simulink model "PMS_Motor_level2"  (Simulink 6.4)
settings: Solver=FixedStepDiscrete  StartTime=0.0  StopTime=0.3  RelTol=1e-3
values from neighbouring files (symbols this model uses):
  DC_voltage = 200    [PMS_Motor_data.m]
  model = 'AM_Sqrt'    [ChangeModel.m]    (also in SelectModel.m = 'MCov_AR')
  Ts = 5e-5    (= 5e-05)    [PMS_Motor_data.m]
libraries: powerlib x12, c28xdmclib x4, simulink x4, tiiqmathlib x3, c281xdspchiplib x2, c2000tgtpreflib x1, powerlib_extras x1
CloseFcn:
  | rtwprivate ssgencode ModelCloseRequest Simple_DC_Motor
settings Model: LastModifiedBy=greith  ProdHWDeviceType=TI C2000
settings DataIOCC: SaveOutput=off  SaveTime=off  SignalLoggingName=DataLog
settings OptimizationCC: OptimizeModelRefInitCode=on  LifeSpan=1
settings DebuggingCC: ReadBeforeWriteMsg=DisableAll  ParameterPrecisionLossMsg=none  StrictBusMsg=ErrorLevel1
settings HardwareCC: ProdBitPerChar=16  ProdBitPerInt=16  ProdIntDivRoundTo=Zero  ProdEndianess=LittleEndian  ProdWordSize=16  ProdHWDeviceType=TI C2000  TargetHWDeviceType=32-bit Generic
settings RTWCC: SystemTargetFile=ti_c2000_ert.tlc  GenCodeOnly=on  TemplateMakefile=ti_c2000_ert.tmf  Description=Embedded Target for TI C2000 DSP (ERT)  GenerateReport=on  ProcessScript=ti_c2000_ert_make_rtw_hook  IncludeHyperlinkInReport=on  LaunchReport=on
settings CodeAppCC: IgnoreCustomStorageClasses=off
settings STFCustomTargetCC: TargetFcnLib=ansi_tfl_tmw.mat  GenFloatMathFcnCalls=ANSI_C  ModelReferenceCompliant=off  CombineOutputUpdateFcns=on  IncludeERTFirstTime=on  ERTCustomFileBanners=on  SystemTargetFile=ti_c2000_ert.tlc
settings ERTTargetCC: TargetFcnLib=ansi_tfl_tmw.mat  GenFloatMathFcnCalls=ANSI_C  ModelReferenceCompliant=off  IncludeERTFirstTime=on  ERTFirstTimeCompliant=off  SupportContinuousTime=on  SupportNonInlinedSFcns=on  InlinedParameterPlacement=NonHierarchical  ERTCustomFileTemplate=example_file_process.tlc  InitialValueSource=Model

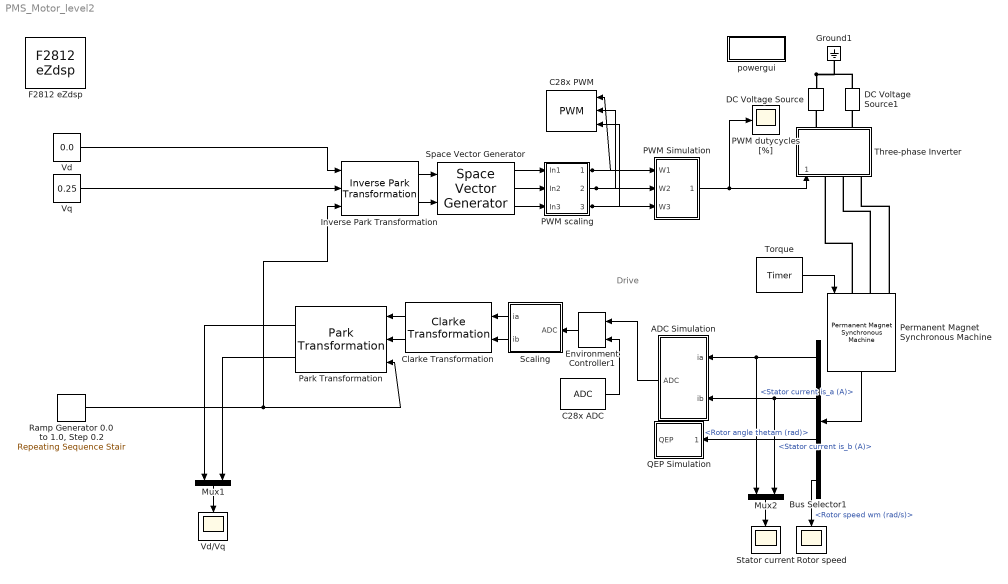
== system PMS_Motor_level2 ==
  note: Drive
  ADC Simulation : Subsystem  Orientation=left
  Bus Selector1 : BusSelector  Orientation=left  OutputSignals=Stator current is_a (A),Stator current is_b (A),Rotor angle thetam (rad),Rotor speed wm (rad/s)
  C28x ADC : c281xdspchiplib/ADC  useModule=A  useMode=Sequential  sourceSOC=Software  Ts=-1  dType=uint16  postInterrupt=off  numConversionsSingle=3  numConversionsDouble=1  conv0=ADCINB0  conv1=ADCINB1  conv2=ADCINB2  conv3=ADCINB3  conv4=ADCINA4  conv5=ADCINA5  conv6=ADCINB6  conv7=ADCINA7  conv8=ADCINB0  conv9=ADCINB1  conv10=ADCINB2  conv11=ADCINB3  conv12=ADCINB4  conv13=ADCINB5  conv14=ADCINB6  conv15=ADCINB7  convAB0=ADCINA0 and ADCINB0  convAB1=ADCINA1 and ADCINB1  convAB2=ADCINA5 and ADCINB5  convAB3=ADCINA1 and ADCINB1  convAB4=ADCINA1 and ADCINB1  convAB5=ADCINA1 and ADCINB1  convAB6=ADCINA1 and ADCINB1  convAB7=ADCINA1 and ADCINB1  convA0=ADCINA0  convA1=ADCINA1  convA2=ADCINA7  convA3=ADCINA3  convA4=ADCINA4  convA5=ADCINA5  convA6=ADCINA6  convA7=ADCINA7  convB0=ADCINB0  convB1=ADCINB1  convB2=ADCINB2  convB3=ADCINB3  convB4=ADCINB4  convB5=ADCINB5  convB6=ADCINB6  convB7=ADCINB7  c28xmultiPort=off
  C28x PWM : c281xdspchiplib/PWM  Orientation=left  useModule=A  timerSource=Specify via dialog  timerPeriod=(2^12)+1  waveformType=Symmetric  periodUnits=Clock cycles  unit1Status=on  unit1Source=Input port  unit1Value=4096  unit2Status=on  unit2Source=Input port  unit2Value=4096  unit3Status=on  unit3Source=Input port  unit3Value=4096  dutyCycleUnits=Clock cycles  logicSource=Specify via dialog  unit1_1Logic=Active high  unit1_2Logic=Active low  unit2_1Logic=Active high  unit2_2Logic=Active low  unit3_1Logic=Active high  unit3_2Logic=Active low  enableDeadband1=on  enableDeadband2=on  enableDeadband3=on  deadbandPrescaler=8  deadbandPeriodSource=Specify via dialog  deadbandPeriod=15  adcstartEvent=None
  Clarke Transformation : c28xdmclib/Clarke Transformation  Orientation=left
  DC Voltage Source : powerlib/Electrical Sources/DC Voltage Source  Orientation=down  SystemSampleTime=-1  Amplitude=DC_voltage  Measurements=None
  DC Voltage Source1 : powerlib/Electrical Sources/DC Voltage Source  Orientation=up  SystemSampleTime=-1  Amplitude=DC_voltage  Measurements=None
  Environment Controller1 : simulink/Signal Routing/Environment Controller  Orientation=left  SystemSampleTime=-1
  F2812 eZdsp : c2000tgtpreflib/F2812 eZdsp  Tag=C2000 TARGET PREFERENCES BLOCK  SystemSampleTime=-1
  Ground1 : powerlib/Elements/Ground  Orientation=up  PhysicalDomain=powersysdomain  SubClassName=unknown  LeftPortType=p1  RightPortType=p1  LConnTagsString=a
  Inverse Park Transformation : c28xdmclib/Inverse Park Transformation
  Mux1 : Mux  Orientation=down  Inputs=2
  Mux2 : Mux  Orientation=down  Inputs=2
  PWM Simulation : Subsystem
  PWM dutycycles [%] : Scope
      settings: TimeRange=1.8  YMin=0.35  YMax=0.625  SaveName=ScopeData4
  PWM scaling : Subsystem
  Park Transformation : c28xdmclib/Park Transformation  Orientation=left
  Permanent Magnet Synchronous Machine : powerlib/Machines/Permanent Magnet Synchronous Machine  Orientation=down  SystemSampleTime=-1  FluxDistribution=Sinusoidal  MechanicalLoad=Torque Tm  PresetModel=No  ShowDetailedParameters=on  Resistance=1.6  Inductance=8.5e-3  dqInductances=[0.006365 0.006365]  Flux=0.1852  Flat=120  Mechanical=[0.0001854 5.396e-005 1]
  QEP Simulation : Subsystem  Orientation=left
  "Ramp Generator 0.0 to 1.0, Step 0.2" : simulink/Sources/Repeating Sequence Stair  SystemSampleTime=-1  OutValues=[0.0:0.0005:1.0]  tsamp=0.00005  OutputDataTypeScalingMode=Specify via dialog  OutDataType=sfix(32)  ConRadixGroup=Use Specified Scaling  OutScaling=2^-17
  Rotor speed : Scope
      settings: Orientation=down  TimeRange=4.5  YMin=-150  YMax=1000
  Scaling : Subsystem  Orientation=left
  Space Vector Generator : c28xdmclib/Space Vector Generator
  Stator current : Scope
      settings: Orientation=down  TimeRange=0.5567010309278351  YMin=0  YMax=4000  SaveName=ScopeData6
  Three-phase Inverter : Subsystem  Orientation=up  AncestorBlock=AC2DriveInternalModels/Three-phase Inverter (average model)  mask(SPSdrives Converter){Device=IGBT / Diodes, SnubberResistance=500, SnubberCapacitance=1e-9, Ron=1e-3, ForwardVoltages=[1.2,1.2], GTOparameters=[10e-6,20e-6], IGBTparameters=[1e-6,2e-6], converterType=Inverter}
      mask prompts: SnubberResistance "Snubber resistance Rs (Ohms)"; SnubberCapacitance "Snubber capacitance Cs (F)"; Ron "Ron (Ohms)"; ForwardVoltages "Forward voltages  [ Device Vf(V) , Diode Vfd(V)]"; GTOparameters "GTO parameters"; IGBTparameters "[  Tf (s) , Tt (s)  ]"; converterType "Converter type:"
      mask help: This block represents an average-value three-phase inverter. "Duty" contains the duty cycles [alpha_a,alpha_b,alpha_c] of the three inverter arms.
      mask StyleString: popup(Diodes|Thyristors|GTO / Diodes|MOSFET / Diodes|IGBT / Diodes|Ideal Switches),edit,edit,edit,edit,edit,edit,popup(Rectifier|Inverter)
      mask Display: plot(0,0,100,100,[39 39 23.8],[71 28 28],[44 56 49.6 56 52.8 56 61 61],[39.2 33.6 32.8 33.6 40.8 33.6 30 12.4],[44 44 44 61 61],[28 71 60 66.4 90],[75 67 83 75 67 83 75 75],[54 42 42 54 54 54 54 66],[61 75 75],[24 24 42],[75 75 61],[66,76,76])
  Torque : powerlib_extras/Control  Blocks/Timer  SystemSampleTime=-1  t=[0 5]  e=[-5 5]
  Vd : Constant  Value=0.0  OutDataTypeMode=Specify via dialog  OutDataType=sfix(32)  ConRadixGroup=Use specified scaling  OutScaling=2^-17  SampleTime=inf  FramePeriod=inf
  Vd/Vq : Scope
      settings: Orientation=down  TimeRange=0.5567010309278351  YMin=0  YMax=4000
  Vq : Constant  Value=0.25  OutDataTypeMode=Specify via dialog  OutDataType=sfix(32)  ConRadixGroup=Use specified scaling  OutScaling=2^-17  SampleTime=inf  FramePeriod=inf
  powergui : Subsystem  AncestorBlock=powerlib/powergui  InitFcn=|  mask(PSB option menu block){SimulationMode=Discrete, SampleTime=5e-5, echomessages=off, x0status=blocks, Frange=[0:2:500], Ylog=off, Xlog=on, ShowGrid=off, save=off, variable=ZData, structure=, ZoomFFT=on, StartTime=0.0, cycles=1, DisplayStyle=1, fundamental=60, FreqAxis=off, MaxFrequency=1000, frequencyindice=1, frequencyindicesteady=1, RmsSteady=1, display=off, Ts=0, frequency=60, methode=off}
      | powerguiblock = gcb;                                        
      | blk = get_param(powerguiblock,'blocks');                    
      | NbBlocks = length(blk);                                     
      | if NbBlocks>2                                               
      | % clean-up:                                                 
      | for m=1:NbBlocks-2                                          
      | delete_block([powerguiblock,'/EquivalentModel',num2str(m)]);
      | end                                                         
      | end
      mask prompts: SimulationMode "General parameter: Simulation Mode"; SampleTime "General parameter: Sample Time"; echomessages "General parameter: Echo  Messages"; x0status "Initial electrical states status"; Frange "Impedance tool: Frequency Range"; Ylog "Impedance tool: Log impedance"; Xlog "Impedance tool: log Frequency"; ShowGrid "Impedance tool: grid"; save "Impedance tool: Save Data To Workspace"; variable "Impedance tool: Variable Name"; structure "Structure Name (PSBFFTSCOPE)"; ZoomFFT "ZoomFFT (PSBFFTSCOPE)"; StartTime "Start Time (PSBFFTSCOPE)"; cycles "Cycles (PSBFFTSCOPE)"; DisplayStyle "Display style (PSBFFTSCOPE)"; fundamental "Fundamental (PSBFFTSCOPE)"; FreqAxis "Frequency Axis (PSBFFTSCOPE)"; MaxFrequency "Max Frequency (PSBFFTSCOPE)"; frequencyindice "Frequency indice  (PSBLOADFLOW)"; frequencyindicesteady "Frequency indice (STEADYSTATE)"; RmsSteady "RMS display (STEADYSTATE)"; display "Display Results"; Ts "Sample time (s):"; frequency "General parameter: phasor frequency"; methode "Phasor simulation"
      mask init:
      | powerlibroot = which('powersysdomain');
      | PSBroot = powerlibroot(1:end-16);
      | %
      | switch SimulationMode
      | 	case 1
      | 		message=sprintf('Continuous');
      | 	case 2
      |         message=sprintf('Discrete,\nTs = %.4g s.',SampleTime);
      | 	case 3
      | 		message=sprintf('Phasors');
      | end
      | if strcmp(bdroot,'powerlib')
      |   message='powergui';
      | end
      | power_initmask();
      settings: CopyFcn=powergui('Copy_Callback',gcb,0,[]);  DeleteFcn=powergui('Copy_Callback',gcb,1,[]);powergui('Close_Callback',gcb,[],[]);  ModelCloseFcn=powergui('Close_Callback',gcb,[],[]);  NameChangeFcn=handles = get_param(gcb,'UserData');if ~isempty(handles);delete(handles.powergui);end
      settings: PreSaveFcn=|
      | %try
      | %close(get_param(gcbh,'userdata'))
      | %end
      | 
      | powergui('Close_Callback',gcb,[],[]);
      settings: OpenFcn=|
      | if (power_openblockproxy ('secondary'))
      | powergui(gcb,'PM')
      | end;
      mask Help: web(psbhelp)
      mask StyleString: popup(Continuous|Discrete|Phasor),edit,checkbox,popup(blocks|steady|zero),edit,checkbox,checkbox,checkbox,checkbox,edit,edit,checkbox,edit,edit,edit,edit,checkbox,edit,edit,edit,edit,checkbox,edit,edit,checkbox
      mask Display: disp(message)
  wires:
  Inverse Park Transformation/1 -> Space Vector Generator/1
  Inverse Park Transformation/2 -> Space Vector Generator/2
  Space Vector Generator/1 -> PWM scaling/1(In1)
  Space Vector Generator/2 -> PWM scaling/2(In2)
  Space Vector Generator/3 -> PWM scaling/3(In3)
  PWM scaling/1(Out1) -> C28x PWM/1, PWM Simulation/1(W1)
  PWM scaling/2(Out2) -> C28x PWM/2, PWM Simulation/2(W2)
  PWM scaling/3(Out3) -> C28x PWM/3, PWM Simulation/3(W3)
  Vd/1 -> Inverse Park Transformation/1
  Vq/1 -> Inverse Park Transformation/2
  "Ramp Generator 0.0 to 1.0, Step 0.2"/1 -> Inverse Park Transformation/3, Park Transformation/3
  PWM Simulation/1(Duty) -> Three-phase Inverter/1(Duty), PWM dutycycles [%]/1
  Bus Selector1/1 -> ADC Simulation/1(ia), Mux2/1  "<Stator current is_a (A)>"
  Bus Selector1/2 -> ADC Simulation/2(ib), Mux2/2  "<Stator current is_b (A)>"
  Bus Selector1/3 -> QEP Simulation/1(angle)  "<Rotor angle thetam (rad)>"
  Permanent Magnet Synchronous Machine/1 -> Bus Selector1/1
  Torque/1 -> Permanent Magnet Synchronous Machine/1
  Bus Selector1/4 -> Rotor speed/1  "<Rotor speed wm (rad/s)>"
  Mux2/1 -> Stator current/1
  Mux1/1 -> Vd/Vq/1
  ADC Simulation/1(ADC) -> Environment Controller1/1
  C28x ADC/1 -> Environment Controller1/2
  Environment Controller1/1 -> Scaling/1(ADC)
  Scaling/1(ia) -> Clarke Transformation/1
  Scaling/2(ib) -> Clarke Transformation/2
  Clarke Transformation/1 -> Park Transformation/1
  Clarke Transformation/2 -> Park Transformation/2
  Park Transformation/1 -> Mux1/1
  Park Transformation/2 -> Mux1/2
  connections:
  DC Voltage Source/LConn1 -- Ground1/LConn1 -- DC Voltage Source1/RConn1
  Three-phase Inverter/RConn2 -- DC Voltage Source1/LConn1
  Three-phase Inverter/RConn1 -- DC Voltage Source/RConn1
  Permanent Magnet Synchronous Machine/LConn1 -- Three-phase Inverter/LConn1
  Permanent Magnet Synchronous Machine/LConn2 -- Three-phase Inverter/LConn2
  Permanent Magnet Synchronous Machine/LConn3 -- Three-phase Inverter/LConn3

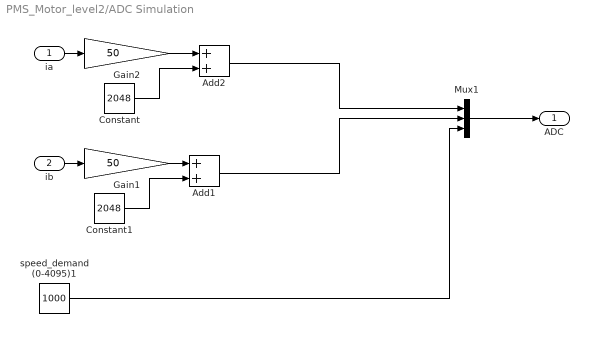
== system PMS_Motor_level2/ADC Simulation ==
  ia : Inport
  ib : Inport  Port=2
  Add1 : Sum  OutDataTypeMode=uint16  OutScaling=2^-10
  Add2 : Sum  OutDataTypeMode=uint16  OutScaling=2^-10
  Constant : Constant  Value=2048  OutDataTypeMode=uint16  OutDataType=sfix(16)  ConRadixGroup=Use specified scaling  OutScaling=2^0  SampleTime=inf  FramePeriod=inf
  Constant1 : Constant  Value=2048  OutDataTypeMode=uint16  OutDataType=sfix(16)  ConRadixGroup=Use specified scaling  OutScaling=2^0  SampleTime=inf  FramePeriod=inf
  Gain1 : Gain  Gain=50  OutDataType=uint(16)
  Gain2 : Gain  Gain=50  OutDataType=uint(16)
  Mux1 : Mux  Inputs=3
  speed_demand (0-4095)1 : Constant  Value=1000  OutDataTypeMode=uint16  OutDataType=sfix(16)  ConRadixGroup=Use specified scaling  OutScaling=2^0  SampleTime=inf  FramePeriod=inf
  ADC : Outport
  wires:
  ia/1 -> Gain2/1
  Constant/1 -> Add2/2
  Constant1/1 -> Add1/2
  ib/1 -> Gain1/1
  Gain2/1 -> Add2/1
  Gain1/1 -> Add1/1
  Add1/1 -> Mux1/2
  Add2/1 -> Mux1/1
  speed_demand (0-4095)1/1 -> Mux1/3
  Mux1/1 -> ADC/1

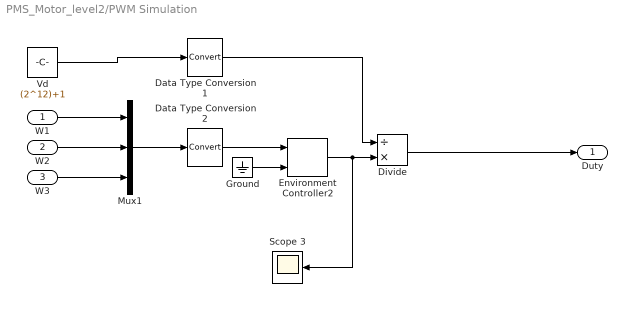
== system PMS_Motor_level2/PWM Simulation ==
  W1 : Inport
  W2 : Inport  Port=2
  W3 : Inport  Port=3
  Data Type Conversion1 : DataTypeConversion  OutDataTypeMode=double
  Data Type Conversion2 : DataTypeConversion  OutDataTypeMode=double
  Divide : Product  Inputs=/*  OutScaling=2^-10
  Environment Controller2 : simulink/Signal Routing/Environment Controller  SystemSampleTime=-1
  Ground : Ground
  Mux1 : Mux  Inputs=3
  Scope 3 : Scope
      settings: TimeRange=0.05820879566685688  YMin=700  YMax=1175  SaveName=ScopeData2
  Vd : Constant  Value=(2^12)+1  OutDataTypeMode=double  OutDataType=sfix(32)  ConRadixGroup=Use specified scaling  OutScaling=2^-17  SampleTime=inf  FramePeriod=inf
  Duty : Outport
  wires:
  Ground/1 -> Environment Controller2/2
  Mux1/1 -> Data Type Conversion2/1
  Environment Controller2/1 -> Scope 3/1, Divide/2
  Divide/1 -> Duty/1
  W1/1 -> Mux1/1
  W2/1 -> Mux1/2
  W3/1 -> Mux1/3
  Data Type Conversion1/1 -> Divide/1
  Data Type Conversion2/1 -> Environment Controller2/1
  Vd/1 -> Data Type Conversion1/1

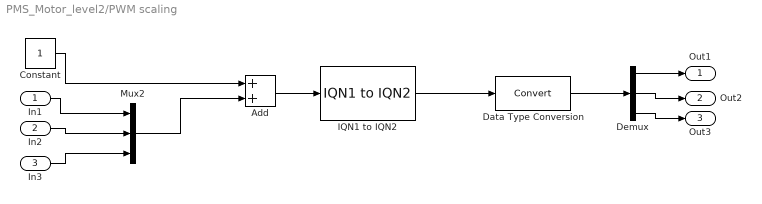
== system PMS_Motor_level2/PWM scaling ==
  In1 : Inport
  In2 : Inport  Port=2
  In3 : Inport  Port=3
  Add : Sum  OutScaling=2^-10
  Constant : Constant  Value=1  OutDataTypeMode=Specify via dialog  OutDataType=sfix(32)  ConRadixGroup=Use specified scaling  OutScaling=2^-17  SampleTime=inf  FramePeriod=inf
  Data Type Conversion : DataTypeConversion  OutDataTypeMode=uint16  ConvertRealWorld=Stored Integer (SI)
  Demux : Demux  Outputs=3
  IQN1 to IQN2 : tiiqmathlib/IQN1 to IQN2  New_Q=11
  Mux2 : Mux  Inputs=3
  Out1 : Outport
  Out2 : Outport  Port=2
  Out3 : Outport  Port=3
  wires:
  In1/1 -> Mux2/1
  Add/1 -> IQN1 to IQN2/1
  Constant/1 -> Add/1
  IQN1 to IQN2/1 -> Data Type Conversion/1
  In3/1 -> Mux2/3
  In2/1 -> Mux2/2
  Mux2/1 -> Add/2
  Data Type Conversion/1 -> Demux/1
  Demux/3 -> Out3/1
  Demux/2 -> Out2/1
  Demux/1 -> Out1/1

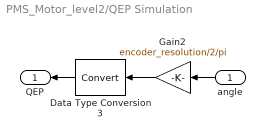
== system PMS_Motor_level2/QEP Simulation ==
  angle : Inport  Orientation=left
  Data Type Conversion3 : DataTypeConversion  Orientation=left  OutDataTypeMode=uint16  OutDataType=sfix(32)  OutScaling=2^-24  SampleTime=Ts
  Gain2 : Gain  Orientation=left  Gain=encoder_resolution/2/pi  OutDataTypeMode=Specify via dialog  OutDataType=uint(16)
  QEP : Outport  Orientation=left
  wires:
  Gain2/1 -> Data Type Conversion3/1
  Data Type Conversion3/1 -> QEP/1
  angle/1 -> Gain2/1

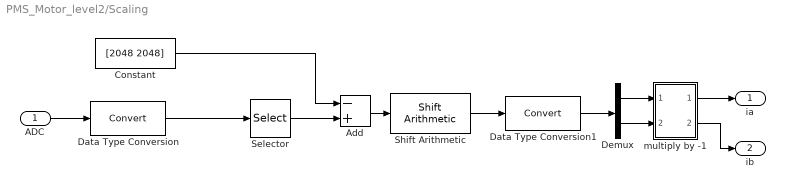
== system PMS_Motor_level2/Scaling ==
  ADC : Inport
  Add : Sum  Inputs=-+  OutScaling=2^-10
  Constant : Constant  Value=[2048 2048]  OutDataTypeMode=int32  OutDataType=sfix(32)  ConRadixGroup=Use specified scaling  OutScaling=2^-12  SampleTime=inf  FramePeriod=inf
  Data Type Conversion : DataTypeConversion  OutDataTypeMode=int32  OutDataType=sfix(32)  OutScaling=2^-12  ConvertRealWorld=Stored Integer (SI)
  Data Type Conversion1 : DataTypeConversion  OutDataTypeMode=Specify via dialog  OutDataType=sfix(32)  OutScaling=2^-17  ConvertRealWorld=Stored Integer (SI)
  Demux : Demux  Outputs=2
  Selector : Selector  Elements=[1 2]  InputPortWidth=3
  Shift Arithmetic : simulink/Logic and Bit Operations/Shift Arithmetic  SystemSampleTime=-1  nBitShiftRight=-6  nBinPtShiftRight=0
  multiply by -1 : Subsystem
  ia : Outport
  ib : Outport  Port=2
  wires:
  ADC/1 -> Data Type Conversion/1
  multiply by -1/2(Out2) -> ib/1
  multiply by -1/1(Out1) -> ia/1
  Demux/2 -> multiply by -1/2(In2)
  Demux/1 -> multiply by -1/1(In1)
  Data Type Conversion1/1 -> Demux/1
  Shift Arithmetic/1 -> Data Type Conversion1/1
  Add/1 -> Shift Arithmetic/1
  Selector/1 -> Add/2
  Constant/1 -> Add/1
  Data Type Conversion/1 -> Selector/1

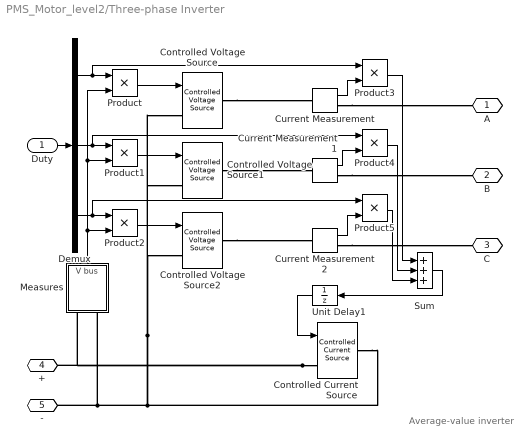
== system PMS_Motor_level2/Three-phase Inverter ==
  note: Average-value inverter
  Duty : Inport
  Controlled Current Source : powerlib/Electrical Sources/Controlled Current Source  SystemSampleTime=-1  Initialize=on  Source_Type=AC  Amplitude=0  Phase=0  Frequency=0  Measurements=None
  Controlled Voltage Source : powerlib/Electrical Sources/Controlled Voltage Source  SystemSampleTime=-1  Initialize=on  Source_Type=AC  Amplitude=0  Phase=0  Frequency=0  Measurements=None
  Controlled Voltage Source1 : powerlib/Electrical Sources/Controlled Voltage Source  SystemSampleTime=-1  Initialize=on  Source_Type=AC  Amplitude=0  Phase=0  Frequency=0  Measurements=None
  Controlled Voltage Source2 : powerlib/Electrical Sources/Controlled Voltage Source  SystemSampleTime=-1  Initialize=on  Source_Type=AC  Amplitude=0  Phase=0  Frequency=0  Measurements=None
  Current Measurement : powerlib/Measurements/Current Measurement  SystemSampleTime=-1  PhasorSimulation=off  OutputType=Complex  PSBequivalent=0
  Current Measurement1 : powerlib/Measurements/Current Measurement  SystemSampleTime=-1  PhasorSimulation=off  OutputType=Complex  PSBequivalent=0
  Current Measurement2 : powerlib/Measurements/Current Measurement  SystemSampleTime=-1  PhasorSimulation=off  OutputType=Complex  PSBequivalent=0
  Demux : Demux  Outputs=3
  Measures : Subsystem  Orientation=up
  Product{,1..5} (6 alike) : Product  SaturateOnIntegerOverflow=on
  Sum : Sum  Inputs=+++  SaturateOnIntegerOverflow=on
  Unit Delay1 : UnitDelay  Orientation=left  SampleTime=Ts
  A : PMIOPort  Orientation=left  Port=1  Side=Left
  B : PMIOPort  Orientation=left  Port=2  Side=Left
  C : PMIOPort  Orientation=left  Port=3  Side=Left
  + : PMIOPort  Port=4  Side=Right
  - : PMIOPort  Port=5  Side=Right
  wires:
  Unit Delay1/1 -> Controlled Current Source/1
  Demux/1 -> Product/1, Product3/1
  Duty/1 -> Demux/1
  Product/1 -> Controlled Voltage Source/1
  Product1/1 -> Controlled Voltage Source1/1
  Product2/1 -> Controlled Voltage Source2/1
  Demux/2 -> Product1/1, Product4/1
  Demux/3 -> Product2/1, Product5/1
  Measures/1(V bus) -> Product/2, Product1/2, Product2/2
  Product3/1 -> Sum/1
  Product4/1 -> Sum/2
  Product5/1 -> Sum/3
  Sum/1 -> Unit Delay1/1
  Current Measurement1/1 -> Product4/2
  Current Measurement/1 -> Product3/2
  Current Measurement2/1 -> Product5/2
  connections:
  Controlled Voltage Source/RConn1 -- Current Measurement/LConn1
  Controlled Voltage Source1/RConn1 -- Current Measurement1/LConn1
  Controlled Voltage Source2/RConn1 -- Current Measurement2/LConn1
  Controlled Current Source/LConn1 -- +/RConn1 -- Measures/LConn1
  Controlled Current Source/RConn1 -- Measures/LConn2 -- -/RConn1 -- Controlled Voltage Source2/LConn1 -- Controlled Voltage Source1/LConn1 -- Controlled Voltage Source/LConn1
  Current Measurement/RConn1 -- A/RConn1
  Current Measurement1/RConn1 -- B/RConn1
  Current Measurement2/RConn1 -- C/RConn1

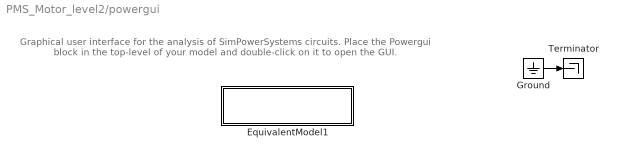
== system PMS_Motor_level2/powergui ==
  note: Graphical user interface for the analysis of  SimPowerSystems circuits.
      | Place the Powergui block in the top-level of your model and double-click
      | on it to open the GUI.
  EquivalentModel1 : Subsystem
      mask init:
      | SPS = get_param(gcbh,'UserData');
      | if isempty(SPS)
      | 	Ts=1;
      |     A=0;
      |     B=0;
      |     C=0;
      |     D=0;
      |     x0=0;
      | else
      | 	A=SPS.Adiscrete;
      |     B=SPS.Bdiscrete;
      |     C=SPS.Cdiscrete;
      |     D=SPS.Ddiscrete;
      |     x0=SPS.x0discrete;
      | 	Ts=SPS.fixedstep;
      | end
      mask Display:
      | color('red')
      | disp('EQUIVALENT CIRCUIT')
  Ground : Ground
  Terminator : Terminator
  wires:
  Ground/1 -> Terminator/1

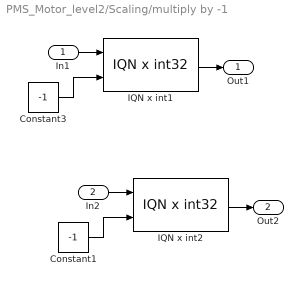
== system PMS_Motor_level2/Scaling/multiply by -1 ==
  In1 : Inport
  In2 : Inport  Port=2
  Constant1 : Constant  Value=-1  OutDataTypeMode=int32  OutDataType=sfix(32)  ConRadixGroup=Use specified scaling  OutScaling=2^-17  SampleTime=inf  FramePeriod=inf
  Constant3 : Constant  Value=-1  OutDataTypeMode=int32  OutDataType=sfix(32)  ConRadixGroup=Use specified scaling  OutScaling=2^-17  SampleTime=inf  FramePeriod=inf
  IQN x int1 : tiiqmathlib/IQN x int32
  IQN x int2 : tiiqmathlib/IQN x int32
  Out1 : Outport
  Out2 : Outport  Port=2
  wires:
  IQN x int2/1 -> Out2/1
  In2/1 -> IQN x int2/1
  Constant1/1 -> IQN x int2/2
  IQN x int1/1 -> Out1/1
  In1/1 -> IQN x int1/1
  Constant3/1 -> IQN x int1/2

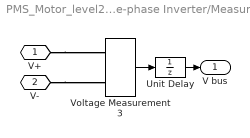
== system PMS_Motor_level2/Three-phase Inverter/Measures ==
  Unit Delay : UnitDelay  SampleTime=Ts
  Voltage Measurement3 : powerlib/Measurements/Voltage Measurement  Tag=PoWeRsYsTeMmEaSuReMeNt  SystemSampleTime=-1  PhasorSimulation=off  OutputType=Complex  PSBequivalent=0
  V+ : PMIOPort  Port=1  Side=Left
  V- : PMIOPort  Port=2  Side=Left
  V bus : Outport
  wires:
  Voltage Measurement3/1 -> Unit Delay/1
  Unit Delay/1 -> V bus/1
  connections:
  V+/RConn1 -- Voltage Measurement3/LConn1
  V-/RConn1 -- Voltage Measurement3/LConn2

== system PMS_Motor_level2/powergui/EquivalentModel1 ==
  Sources : Subsystem
  State-Space : S-Function  FunctionName=sfun_spssw_discc  Parameters=Ts,A, B, C, D, x0
  Yout : Subsystem
  wires:
  Sources/1(u) -> State-Space/1
  State-Space/1 -> Yout/1(v,i)

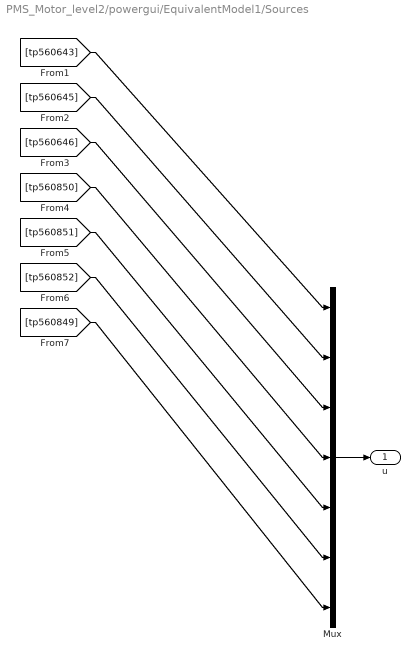
== system PMS_Motor_level2/powergui/EquivalentModel1/Sources ==
  Mux : Mux  Inputs=[2 1 1 1 1 1 1]
  u : Outport
  wires:
  Mux/1 -> u/1
  [tp560643] -> Mux/1
  [tp560645] -> Mux/2
  [tp560646] -> Mux/3
  [tp560850] -> Mux/4
  [tp560851] -> Mux/5
  [tp560852] -> Mux/6
  [tp560849] -> Mux/7

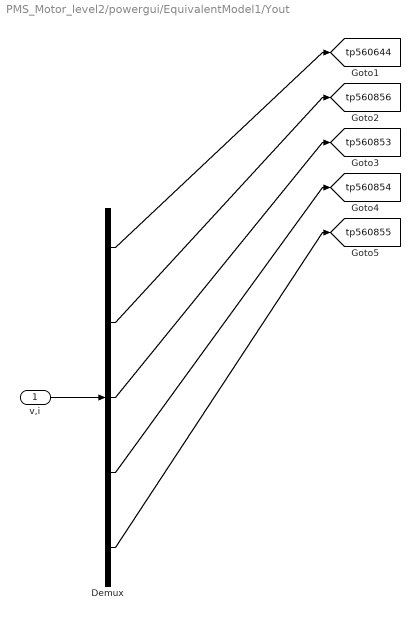
== system PMS_Motor_level2/powergui/EquivalentModel1/Yout ==
  v,i : Inport
  Demux : Demux  Outputs=[2 1 1 1 1]
  tag scope: tp560644=global, tp560853=global, tp560854=global, tp560855=global, tp560856=global
  wires:
  v,i/1 -> Demux/1
  Demux/1 -> [tp560644]
  Demux/2 -> [tp560856]
  Demux/3 -> [tp560853]
  Demux/4 -> [tp560854]
  Demux/5 -> [tp560855]
